simulink model "chap9_4sim"  (Simulink 10.3)
settings: Solver=ode45  StartTime=0.0  StopTime=10  FixedStep=0.00000010  RelTol=1e-3  EnableMultiTasking=on
settings Model: Creator=shipe  LastModifiedBy=shipe  ExtModeTrigMode=oneshot  ExtModeArmWhenConnect=off
settings SolverCC: AlgebraicLoopSolver=Auto
settings DataIOCC: SignalLoggingName=sigsOut
settings OptimizationCC: BooleanDataType=off  ExpressionDepthLimit=128  LifeSpan=auto
settings DebuggingCC: SaveWithParameterizedLinksMsg=none  SignalResolutionControl=TryResolveAllWithWarning  MultiTaskDSMMsg=warning  MultiTaskCondExecSysMsg=none  FcnCallInpInsideContextMsg=error  StateNameClashWarn=none  SFUnexpectedBacktrackingDiag=error  SFNoUnconditionalDefaultTransitionDiag=error  SFExecutionAtInitializationDiag=warning  SFMachineParentedDataDiag=error  ArithmeticOperatorsInVariantConditions=error
settings HardwareCC: TargetUnknown=on
settings SFSimCC: SimUseLocalCustomCode=on  CustomCodeUndefinedFunction=FilterOut
settings RTWCC: RTWUseLocalCustomCode=on
settings CodeAppCC: StateflowObjectComments=off
settings GRTTargetCC: TargetLangStandard=C99 (ISO)
settings ConfigComp: CovExternalEMLEnable=on

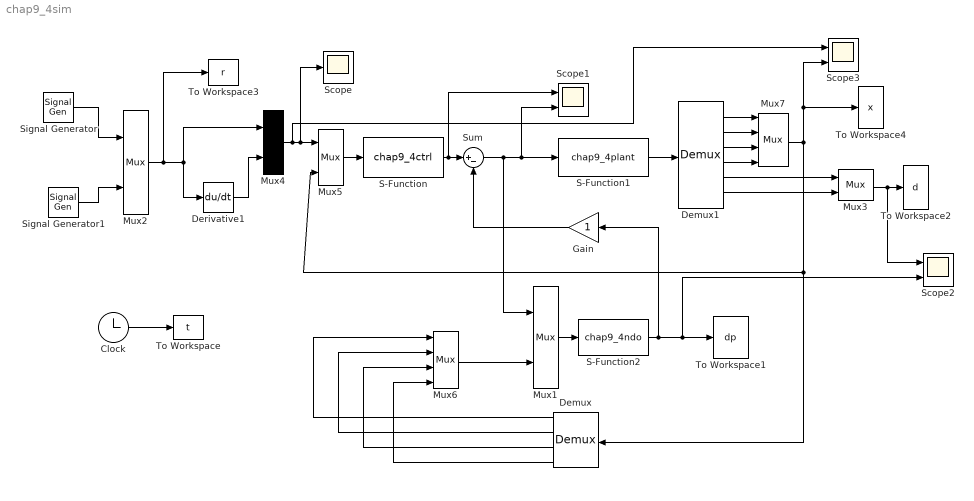
== system chap9_4sim ==
  Clock : Clock
  Demux : Demux
      settings: DisplayOption=none
  Demux1 : Demux  Outputs=6
      settings: DisplayOption=none
  Derivative1 : Derivative
  Gain : Gain  SaturateOnIntegerOverflow=on  OutDataTypeStr=Inherit: Same as input  ParamDataTypeStr=Inherit: Same as input
  Mux{1..5} (5 alike) : Mux  Inputs=2
  Mux6 : Mux
  Mux7 : Mux
  S-Function : S-Function  FunctionName=chap9_4ctrl  SFunctionDeploymentMode=off  EnableBusSupport=off
  S-Function1 : S-Function  FunctionName=chap9_4plant  SFunctionDeploymentMode=off  EnableBusSupport=off
  S-Function2 : S-Function  FunctionName=chap9_4ndo  SFunctionDeploymentMode=off  EnableBusSupport=off
  Scope : Scope
  Scope1 : Scope  NumInputPorts=2
  Scope2 : Scope  NumInputPorts=2
  Scope3 : Scope  NumInputPorts=2
  Signal Generator : SignalGenerator  Frequency=0.1
  Signal Generator1 : SignalGenerator  Frequency=0.1
  Sum : Sum  Inputs=|+-  SaturateOnIntegerOverflow=on
  To Workspace : ToWorkspace  VariableName=t  SampleTime=-1
  To Workspace1 : ToWorkspace  VariableName=dp  SampleTime=-1
  To Workspace2 : ToWorkspace  VariableName=d  SampleTime=-1
  To Workspace3 : ToWorkspace  VariableName=r  SampleTime=-1
  To Workspace4 : ToWorkspace  VariableName=x  SampleTime=-1
  wires:
  Signal Generator/1 -> Mux2/1
  Signal Generator1/1 -> Mux2/2
  Clock/1 -> To Workspace/1
  Mux1/1 -> S-Function2/1
  S-Function2/1 -> Scope2/2, To Workspace1/1, Gain/1
  Mux2/1 -> Derivative1/1, Mux4/1, To Workspace3/1
  Mux5/1 -> S-Function/1
  Mux4/1 -> Scope3/1, Scope/1, Mux5/1
  Derivative1/1 -> Mux4/2
  Mux6/1 -> Mux1/2
  Demux/2 -> Mux6/2
  Demux/1 -> Mux6/1
  Demux/3 -> Mux6/3
  Demux/4 -> Mux6/4
  S-Function1/1 -> Demux1/1
  Demux1/1 -> Mux7/1
  Demux1/2 -> Mux7/2
  Demux1/3 -> Mux7/3
  Demux1/4 -> Mux7/4
  Mux7/1 -> Demux/1, Mux5/2, Scope3/2, To Workspace4/1
  Demux1/5 -> Mux3/1
  Demux1/6 -> Mux3/2
  Mux3/1 -> Scope2/1, To Workspace2/1
  S-Function/1 -> Scope1/1, Sum/1
  Sum/1 -> Scope1/2, S-Function1/1, Mux1/1
  Gain/1 -> Sum/2
